simulink model "ADC_Filter_Compare"  (R2014b)
settings: configuration reference "Embedded_Configuration" (kept outside this file)
PostLoadFcn:
  | c2000demoscallback(1)
model workspace: external: MAT-File C:\Users\Nathan\Desktop\Git\EmbeddedCoderC2000\FirstCode\Embedded_Config.mat (data not in the file)
undefined symbols (not defined in the file or in its folder): alpha, fdesignblkfcn, gcbh
settings Model: Creator=The MathWorks Inc.  LastModifiedBy=Nathan

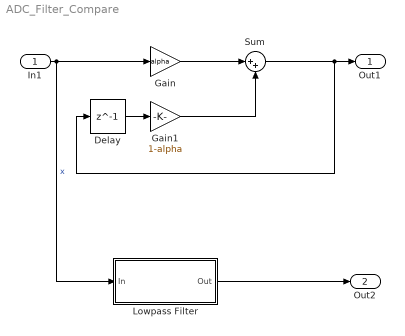
== system ADC_Filter_Compare ==
  In1 : Inport  SampleTime=.0001
  Delay : Delay  DelayLength=1
  Gain : Gain  Gain=alpha
  Gain1 : Gain  Gain=1-alpha
  Lowpass Filter : Subsystem  DialogController=fdesignblkfcn  InitFcn=fdesignblkfcn(gcbh, {'InitFcn'});  mask(Lowpass Filter){}
      mask help: Design a lowpass filter
      settings: CopyFcn=fdesignblkfcn(gcbh, {'CopyFcn'});
      mask Help: helpview(mapfilelocation('dsp'), 'dsplowpassfilter');
      mask Display: disp('Lowpass')
  Sum : Sum  Inputs=|++
  Out1 : Outport
  Out2 : Outport  Port=2
  wires:
  In1/1 -> Lowpass Filter/1(In), Gain/1  "x"
  Gain/1 -> Sum/1
  Delay/1 -> Gain1/1
  Gain1/1 -> Sum/2
  Sum/1 -> Delay/1, Out1/1
  Lowpass Filter/1(Out) -> Out2/1

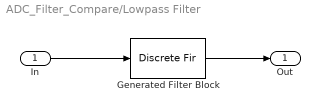
== system ADC_Filter_Compare/Lowpass Filter ==
  In : Inport
  Generated Filter Block : DiscreteFir  Tag=BlockMethodSubSystem  Coefficients=[0.037428405355821877 0.1538393652215066 0.28030240595639061 0.28030240595639061 0.1538393652215066 0.037428405355821877]  InputProcessing=Columns as channels (frame based)
  Out : Outport
  wires:
  In/1 -> Generated Filter Block/1
  Generated Filter Block/1 -> Out/1
